simulink model "MySimModel"  (R2024b)
settings: Solver=VariableStepAuto  StartTime=0.0  StopTime=10.0  RelTol=1e-3
undefined symbols (not defined in the file): DiscIntNeverNeededParam
settings Model: Creator=xinxing  LastModifiedBy=xinxing

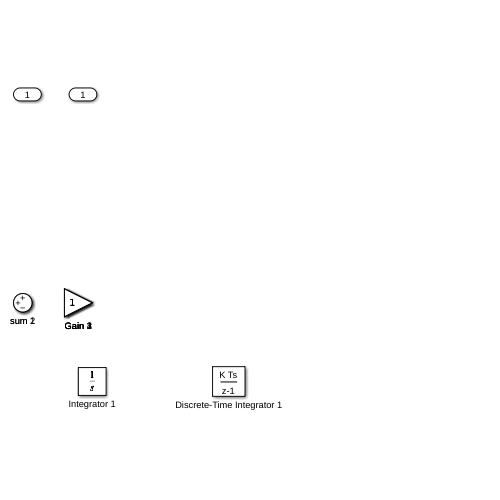
[thumbnail: Simulink's stored preview of the top-level diagram]
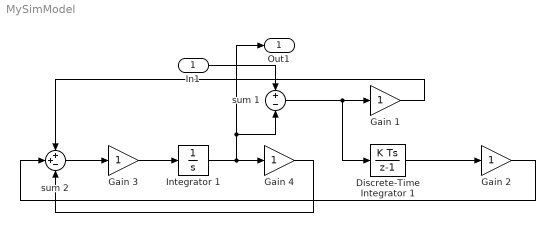
== system MySimModel ==
  In1 : Inport
  Discrete-Time Integrator 1 : DiscreteIntegrator  SampleTime=-1  ICPrevOutput=DiscIntNeverNeededParam  ICPrevScaledInput=DiscIntNeverNeededParam
  Gain {1..4} (4 alike) : Gain
  Integrator 1 : Integrator
  sum 1 : Sum  Inputs=+-
  sum 2 : Sum  Inputs=++-
  Out1 : Outport
  wires:
  Discrete-Time Integrator 1/1 -> Gain 2/1
  Integrator 1/1 -> Out1/1, sum 1/2, Gain 4/1
  sum 1/1 -> Discrete-Time Integrator 1/1, Gain 1/1
  In1/1 -> sum 1/1
  Gain 2/1 -> sum 2/2
  Gain 3/1 -> Integrator 1/1
  Gain 1/1 -> sum 2/1
  Gain 4/1 -> sum 2/3
  sum 2/1 -> Gain 3/1
